simulink model "Motor_Control"  (R2025a)
settings: Solver=VariableStepAuto  StartTime=0.0  StopTime=100  RelTol=1e-3
libraries: simulink x3, mcbcontrolslib x1, mcbplantlib x1, autolibpmsminterior x1
settings Model: SimulationMode=accelerator  Creator=mac  LastModifiedBy=mac

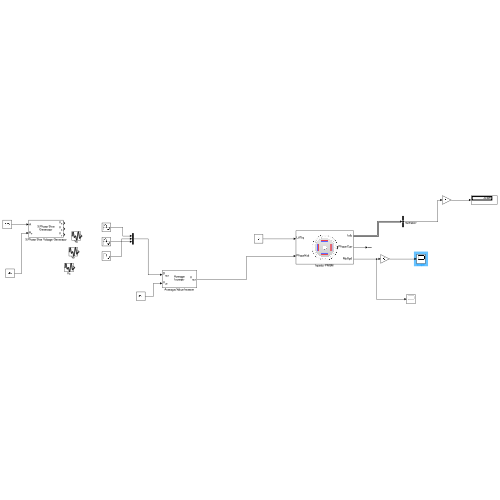
[thumbnail: Simulink's stored preview of the top-level diagram]
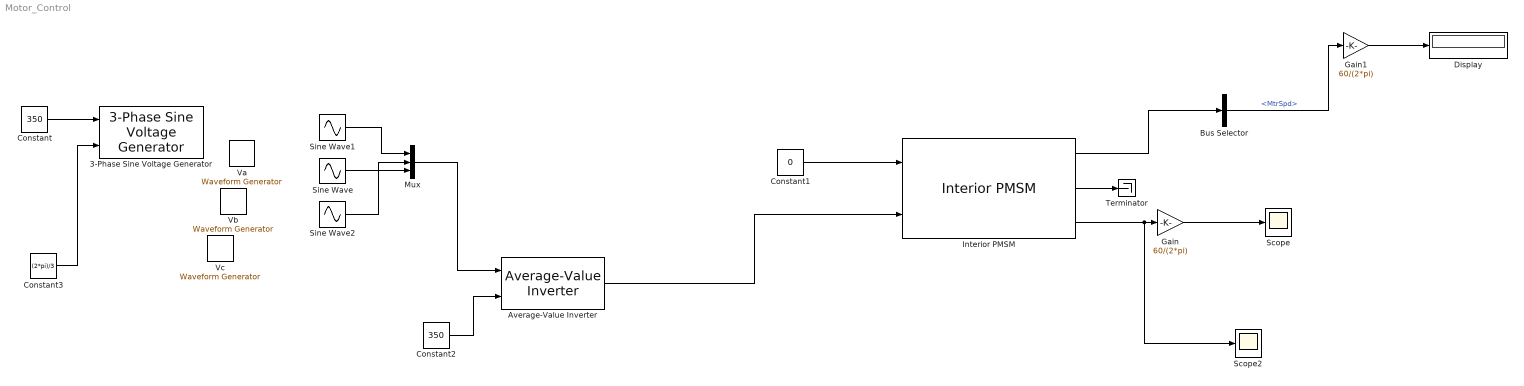
== system Motor_Control ==
  3-Phase Sine Voltage Generator : mcbcontrolslib/3-Phase Sine Voltage Generator  AngleInput=Radians  N_points=1024
      settings: LibrarySourceBlock=mcblib/Controls/Math Transforms/3-Phase Sine Voltage Generator
  Average-Value Inverter : mcbplantlib/Average-Value Inverter
      settings: LibrarySourceBlock=mcblib/Electrical Systems/Inverters/Average-Value Inverter
  Bus Selector : BusSelector  OutputSignals=MtrSpd
  Constant : Constant  Value=350  SampleTime=0.1
  Constant1 : Constant  Value=0  SampleTime=0.1
  Constant2 : Constant  Value=350  SampleTime=0.1
  Constant3 : Constant  Value=(2*pi)/3  SampleTime=0.1
  Display : Display
  Gain : Gain  Gain=60/(2*pi)
  Gain1 : Gain  Gain=60/(2*pi)
  Interior PMSM : autolibpmsminterior/Interior PMSM  port_config=Torque  sim_type=Continuous  Ts=0.1  FilePath=interiorpmsm_motordata.m  P=4  Rs=.2  Ldq=[3.752e-4 4.148e-4]  KConstText=Permanent flux linkage constant (lambda_pm):  lambda_pm=0.1194  Ke=159.9771  mechanical=[0.0027, 4.924e-4, 0]  idq0=[0 0]  theta_init=0  omega_init=0  KConst=0.1194  lambda_pm_calc=0.1194  Kt=1.323  RefBlkName='autolibpmsminterior/Interior PMSM'  aMode=1
      settings: LibrarySourceBlock=autolibemachines/Interior PMSM
  Mux : Mux  Inputs=3
  Scope : Scope
      settings: ActiveDisplayYMinimum=-21100.007629923279  ActiveDisplayYMaximum=23405.736980520905
  Scope2 : Scope
      settings: ActiveDisplayYMinimum=-4904.4126380433927  ActiveDisplayYMaximum=4589.046975035516  DataLoggingVariableName=ScopeData2
  Sine Wave : Sin  Frequency=60  Phase=(2*pi)/3  SampleTime=0.1
  Sine Wave1 : Sin  Frequency=60  SampleTime=0.1
  Sine Wave2 : Sin  Frequency=60  Phase=(4*pi)/3  SampleTime=0.1
  Terminator : Terminator
  Va : simulink/Sources/Waveform Generator  OutMin=[]  OutMax=[]  OutDataTypeStr=double  SelectedSignal=1  Signals=sin(350, 50, 0)  BlockNames=MultiportSwitch_b39b1732653c4ff  SampleTime=0.1
  Vb : simulink/Sources/Waveform Generator  OutMin=[]  OutMax=[]  OutDataTypeStr=double  SelectedSignal=1  Signals=sin(350, 50, 120)  BlockNames=MultiportSwitch_cdfe818d6e4b4fe  SampleTime=0.1
  Vc : simulink/Sources/Waveform Generator  OutMin=[]  OutMax=[]  OutDataTypeStr=double  SelectedSignal=1  Signals=sin(350, 50, 240)  BlockNames=MultiportSwitch_03c28a98a59744a  SampleTime=0.1
  wires:
  Bus Selector/1 -> Gain1/1  "<MtrSpd>"
  Average-Value Inverter/1 -> Interior PMSM/2
  Constant1/1 -> Interior PMSM/1
  Interior PMSM/3 -> Scope2/1, Gain/1
  Gain/1 -> Scope/1
  Interior PMSM/1 -> Bus Selector/1
  Interior PMSM/2 -> Terminator/1
  Constant/1 -> 3-Phase Sine Voltage Generator/1
  Constant3/1 -> 3-Phase Sine Voltage Generator/2
  Constant2/1 -> Average-Value Inverter/2
  Gain1/1 -> Display/1
  Sine Wave1/1 -> Mux/1
  Sine Wave/1 -> Mux/3
  Sine Wave2/1 -> Mux/2
  Mux/1 -> Average-Value Inverter/1
